simulink model "mpcprueba2"  (R2025a)
settings: Solver=FixedStepAuto  StartTime=0.0  StopTime=inf  FixedStep=0.0201  RelTol=1e-3  EnableMultiTasking=on
values from neighbouring files (symbols this model uses):
  H = G'*Qvec*G+Rvec    [mpcwec 1.m]
  Qvec = blkdiag(Qvec,P)    [mpcwec 1.m]
undefined symbols (not defined in the file or in its folder): F, G, Pc, qc, Sc
settings Model: PacingRate=0.790000  ExtModeTrigDuration=10  Creator=The MathWorks, Inc.  LastModifiedBy=aero
settings SolverCC: AlgebraicLoopSolver=TrustRegion  PositivePriorityOrder=on  AutoInsertRateTranBlk=on  MaxZcPerStep=1.0
settings OptimizationCC: EnhancedBackFolding=on  PassReuseOutputArgsAs=Individual arguments  MaxStackSize=64  OptimizeBlockOrder=speed  DifferentSizesBufferReuse=on  OptimizationCustomize=off  EfficientTunableParamExpr=on
settings DebuggingCC: ParameterPrecisionLossMsg=none  ParameterTunabilityLossMsg=error  UnconnectedInputMsg=warning  UnconnectedOutputMsg=warning  UnconnectedLineMsg=warning  SubsystemReferenceDiagnosticForUnitTest=warning  ArithmeticOperatorsInVariantConditions=warning
settings HardwareCC: ProdBitPerPointer=32.0  ProdBitPerSizeT=32.0  ProdBitPerPtrDiffT=32.0  ProdLargestAtomicInteger=Long  ProdLargestAtomicFloat=Double  ProdWordSize=32.0  ProdLongLongMode=on  ProdHWDeviceType=ARM Compatible->ARM Cortex
settings ModelReferenceCC: EnableRefExpFcnMdlSchedulingChecks=on
settings SFSimCC: MATLABDynamicMemAlloc=off  SimTargetLang=C++  SimDLTargetLibrary=mkl-dnn
settings RTWCC: SystemTargetFile=ert.tlc  HardwareBoard=PX4 Pixhawk 6c  TLCOptions="-aInlineSetEventsForThisBaseRateFcn=TLC_FALSE -aSuppressMultiTaskScheduler=TLC_FALSE  -aRateBasedStepFcn=0"  TemplateMakefile=ert_default_tmf  GenerateReport=on  Toolchain=GNU Tools for PX4 Autopilots  IncludeHyperlinkInReport=on  LaunchReport=on  TargetLang=C++  GenerateTraceInfo=on  GenerateTraceReport=on  GenerateTraceReportSl=on  GenerateTraceReportSf=on  GenerateTraceReportEml=on  GPUComputeCapability=3.5  DLArmComputeVersion=19.05  Description=Embedded Coder
settings CodeAppCC: ForceParamTrailComments=on  IgnoreCustomStorageClasses=off  OperatorAnnotations=on  SimulinkDataObjDesc=on  SFDataObjDesc=on  InsertBlockDesc=on
settings ERTTargetCC: ExtModeTransport=3.0  ExtModeStaticAllocSize=1024.0  InlinedParameterPlacement=Hierarchical

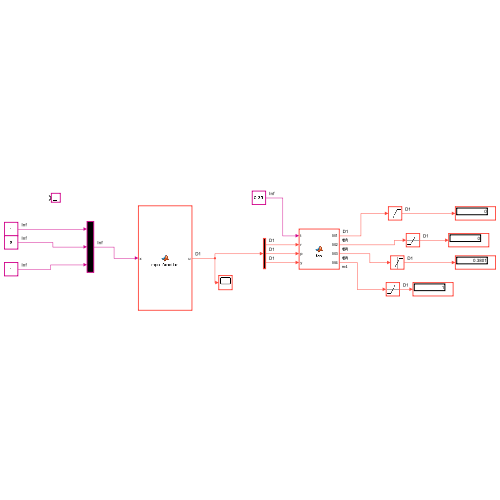
[thumbnail: Simulink's stored preview of the top-level diagram]
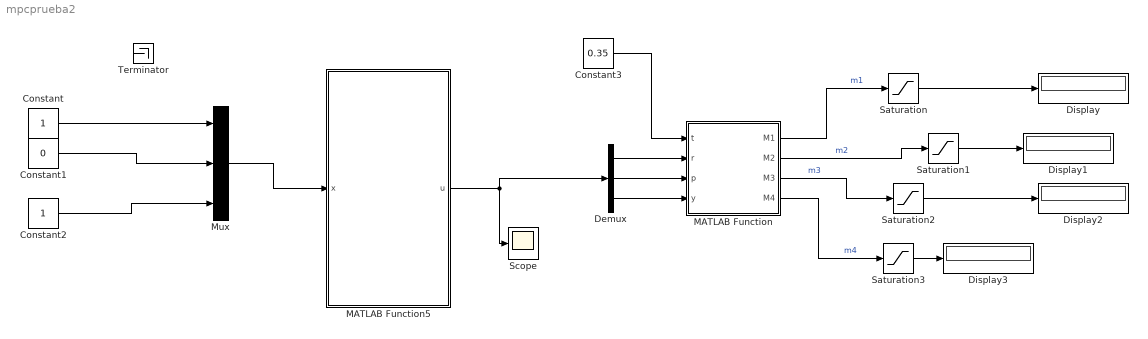
== system mpcprueba2 ==
  Constant : Constant
  Constant1 : Constant  Value=0
  Constant2 : Constant
  Constant3 : Constant  Value=0.35
  Demux : Demux  Outputs=3
  Display{,1..3} (4 alike) : Display
  MATLAB Function : MATLAB Function  TreatAsAtomicUnit=on  SystemSampleTime=0.0201
  MATLAB Function5 : MATLAB Function  TreatAsAtomicUnit=on  SystemSampleTime=0.0201
  Mux : Mux  Inputs=3
  Saturation{,1..3} (4 alike) : Saturate  UpperLimit=1  LowerLimit=0
  Scope : Scope
      settings: ActiveDisplayYMinimum=-1.8561483031737367  ActiveDisplayYMaximum=1.4602099461857099
  Terminator : Terminator
  wires:
  Saturation3/1 -> Display3/1
  Saturation1/1 -> Display1/1
  Saturation2/1 -> Display2/1
  MATLAB Function/2(M2) -> Saturation1/1  "m2"
  Demux/3 -> MATLAB Function/4(y)
  Demux/1 -> MATLAB Function/2(r)
  MATLAB Function5/1(u) -> Demux/1, Scope/1
  MATLAB Function/1(M1) -> Saturation/1  "m1"
  MATLAB Function/4(M4) -> Saturation3/1  "m4"
  Demux/2 -> MATLAB Function/3(p)
  Mux/1 -> MATLAB Function5/1(x)
  Constant3/1 -> MATLAB Function/1(t)
  Saturation/1 -> Display/1
  MATLAB Function/3(M3) -> Saturation2/1  "m3"
  Constant2/1 -> Mux/3
  Constant1/1 -> Mux/2
  Constant/1 -> Mux/1

== matlab function mpcprueba2/MATLAB Function ==
  data: t input; M1 output; r input; p input; y input; M2 output; M3 output; M4 output
function [M1,M2,M3,M4] = fcn(t, r, p, y)
% t: thrust
% r: roll
% p: pitch
% y: yaw

M1 = t - 0.707107*r - 0.707107*p + y;
M2 = t + 0.707107*r + 0.707107*p + y;
M3 = t + 0.707107*r - 0.707107*p - y;
M4 = t - 0.707107*r + 0.707107*p - y;

== matlab function mpcprueba2/MATLAB Function5 ==
  data: x input; u output size=[m 1]; H parameter; F parameter; Qvec parameter; G parameter; Pc parameter; qc parameter; Sc parameter
function u = mpc_function(x, H, F, Qvec, G, Pc, qc, Sc)
persistent opts nu x0
m = 3;
x = double(x);
nu= size(H,1);
x0 = zeros(nu,1,'double');
% uvec = zeros(nu,1);
% === Construcción del QP ===
f = (2*x'*F'*Qvec*G)';

% Resolver QP
opts = optimoptions('quadprog', 'Algorithm','active-set','Display','off');
uvec = quadprog(2*H,f, Pc,qc + Sc*x,[],[],[],[],x0, opts);

% Acción de control (receding horizon)
u = zeros(m,1);
uvec = double(uvec);
u(:) = uvec(1:m);
x0= uvec;
end
